simulink model "BFE_TestHarness"  (Simulink 8.6)
settings: Solver=FixedStepDiscrete  StartTime=0.0  StopTime=3  FixedStep=Ts  RelTol=1e-3
PreLoadFcn:
  | addpath('MBD_Tests')
  | 
  | load('Workspace\EnvVar.mat')
  | run('MBD_Tests\MBD_tests_init.m')
  | if exist('tl_preloadfcn','file'), tl_preloadfcn(gcs,402); end
PostLoadFcn:
  | if exist('tl_postloadfcn','file'), tl_postloadfcn(gcs,402); end
InitFcn:
  | if exist('tlds_init','file'), tlds_init(gcs); end
StartFcn:
  | if exist('tlds_start','file'), tlds_start(gcs); end
StopFcn:
  | if exist('tlds_stop','file'), tlds_stop(gcs); end
undefined symbols (not defined in the file): ddv, Ts, u2, u3, u4
libraries: tllib x11, simulink x8, LIB_TF_G_111 x2, LIB_TF_G_12_StepControl x2, LIB_TF_G_112 x1, LIB_TF_G_113 x1
(part 8 of 17)

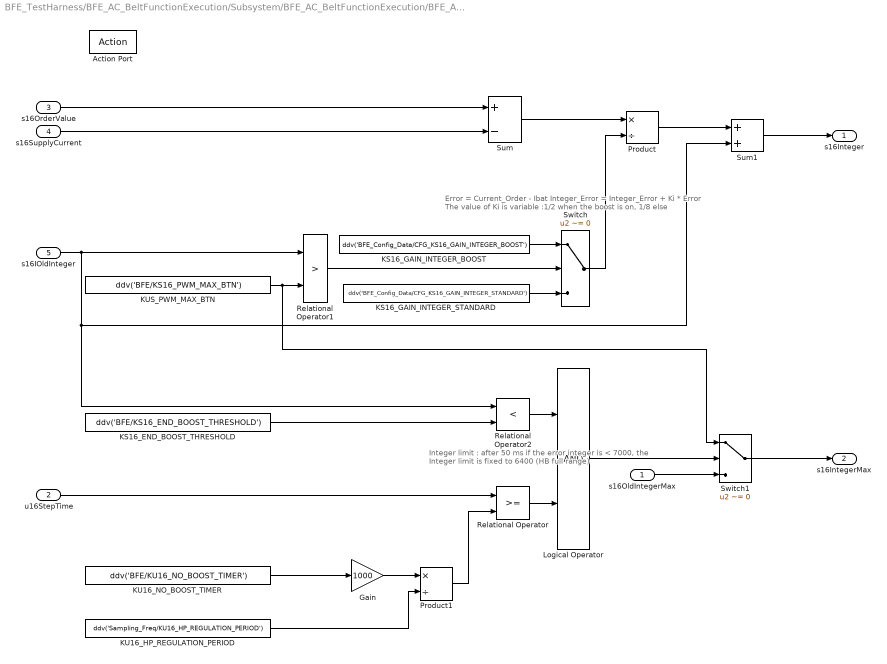
== system BFE_TestHarness/BFE_AC_BeltFunctionExecution/Subsystem/BFE_AC_BeltFunctionExecution/BFE_AC_BeltFunctionExecution/BFE_runExecuteHighPowerStep/HP feature activated/CurrentRegulation/PerformRegulation ==
  note: Error = Current_Order - Ibat
      | Integer_Error = Integer_Error + Ki * Error
      | The value of Ki is variable :1/2 when the boost is on, 1/8 else
  note: Integer limit : after 50 ms if the error integer is < 7000,
      | the Integer limit is fixed to 6400 (HB full range)
  s16OldIntegerMax : Inport  RequirementInfo={} %GIDa_4edf5c18_cfb4_4ed1_aec0_eafae2324e3a
  u16StepTime : Inport  RequirementInfo={} %GIDa_9a24bfd6_4e27_4306_b68d_5ae91b60016c  Port=2
  s16OrderValue : Inport  RequirementInfo={} %GIDa_b1229915_314b_4863_98e3_52cac1c2f91e  Port=3
  s16SupplyCurrent : Inport  RequirementInfo={} %GIDa_425d2a36_5fe9_4dc0_bde3_e336324c322d  Port=4
  s16IOldInteger : Inport  RequirementInfo={} %GIDa_71962a0c_10e9_4e80_9963_0f670b982034  Port=5
  Action Port : ActionPort  RequirementInfo={} %GIDa_15d562f7_52fc_451c_88e4_4cd9eea4c744  ActionType=else
  Gain : Gain  RequirementInfo={} %GIDa_ea57d22b_49e6_4b7f_ac29_28cc2dbba7b3  Gain=1000  OutDataTypeStr=uint16  mask(TL_Gain){data={'output',{'type','UInt16'},'date',735951.66844787041}}
      settings: CopyFcn=if exist('tl_reset_reviewflag','file')==2,tl_reset_reviewflag(gcbh);end  DeleteFcn=if exist('delete_tlblock','file')==2,delete_tlblock(gcbh);end  NameChangeFcn=if exist('rename_tlblock','file')==2,rename_tlblock(gcbh);end  OpenFcn=if exist('tl_open_blockdlg','file')==2,tl_open_blockdlg(gcbh);else,open_system(gcbh,'parameter');end
      mask Help: eval(['if exist(''tl_online_help'',''file'') == 2, tl_online_help(''Topic'',''TL_Gain''),else, web([''jar:file:///'',matlabroot,''/help/toolbox/simulink/help.jar!/slref/' lower(get_param(gcbh,'Blocktype')) '.html''], ''-helpbrowser''),end'])
      mask Display: plot([0, .9, 0],[.05, .5, .95])
  KS16_END_BOOST_THRESHOLD : Constant  RequirementInfo={} %GIDa_f3b0ac08_8bb7_400a_a265_f98ea3ab135f  Value=ddv('BFE/KS16_END_BOOST_THRESHOLD')  OutDataTypeStr=int16  mask(TL_Constant){data={'output',{'variable','BFE/KS16_END_BOOST_THRESHOLD'},'date',735951.66844737274}}
      settings: CopyFcn=if exist('tl_reset_reviewflag','file')==2,tl_reset_reviewflag(gcbh);end  DeleteFcn=if exist('delete_tlblock','file')==2,delete_tlblock(gcbh);end  NameChangeFcn=if exist('rename_tlblock','file')==2,rename_tlblock(gcbh);end  OpenFcn=if exist('tl_open_blockdlg','file')==2,tl_open_blockdlg(gcbh);else,open_system(gcbh,'parameter');end
      mask Help: eval(['if exist(''tl_online_help'',''file'') == 2, tl_online_help(''Topic'',''TL_Constant''),else, web([''jar:file:///'',matlabroot,''/help/toolbox/simulink/help.jar!/slref/' lower(get_param(gcbh,'Blocktype')) '.html''], ''-helpbrowser''),end'])
      mask Display: plot([-0.05, 1.05, NaN, -0.05, 1.05],[.01, .01, NaN, .99, .99])
  KS16_GAIN_INTEGER_BOOST : Constant  RequirementInfo={} %GIDa_006f4594_68bd_400b_90bf_0f2f50455285  Value=ddv('BFE_Config_Data/CFG_KS16_GAIN_INTEGER_BOOST')  OutDataTypeStr=int16  mask(TL_Constant){data={'output',{'variable','BFE_Config_Data/CFG_KS16_GAIN_INTEGER_BOOST'},'date',735951.6684470023}}
      settings: CopyFcn=if exist('tl_reset_reviewflag','file')==2,tl_reset_reviewflag(gcbh);end  DeleteFcn=if exist('delete_tlblock','file')==2,delete_tlblock(gcbh);end  NameChangeFcn=if exist('rename_tlblock','file')==2,rename_tlblock(gcbh);end  OpenFcn=if exist('tl_open_blockdlg','file')==2,tl_open_blockdlg(gcbh);else,open_system(gcbh,'parameter');end
      mask Help: eval(['if exist(''tl_online_help'',''file'') == 2, tl_online_help(''Topic'',''TL_Constant''),else, web([''jar:file:///'',matlabroot,''/help/toolbox/simulink/help.jar!/slref/' lower(get_param(gcbh,'Blocktype')) '.html''], ''-helpbrowser''),end'])
      mask Display: plot([-0.05, 1.05, NaN, -0.05, 1.05],[.01, .01, NaN, .99, .99])
  KS16_GAIN_INTEGER_STANDARD : Constant  RequirementInfo={} %GIDa_e385b7ef_ce71_4760_a7c3_e905cf32e7fa  Value=ddv('BFE_Config_Data/CFG_KS16_GAIN_INTEGER_STANDARD')  OutDataTypeStr=int16  mask(TL_Constant){data={'output',{'variable','BFE_Config_Data/CFG_KS16_GAIN_INTEGER_STANDARD'},'date',735951.66844662034}}
      settings: CopyFcn=if exist('tl_reset_reviewflag','file')==2,tl_reset_reviewflag(gcbh);end  DeleteFcn=if exist('delete_tlblock','file')==2,delete_tlblock(gcbh);end  NameChangeFcn=if exist('rename_tlblock','file')==2,rename_tlblock(gcbh);end  OpenFcn=if exist('tl_open_blockdlg','file')==2,tl_open_blockdlg(gcbh);else,open_system(gcbh,'parameter');end
      mask Help: eval(['if exist(''tl_online_help'',''file'') == 2, tl_online_help(''Topic'',''TL_Constant''),else, web([''jar:file:///'',matlabroot,''/help/toolbox/simulink/help.jar!/slref/' lower(get_param(gcbh,'Blocktype')) '.html''], ''-helpbrowser''),end'])
      mask Display: plot([-0.05, 1.05, NaN, -0.05, 1.05],[.01, .01, NaN, .99, .99])
  KU16_HP_REGULATION_PERIOD : Constant  RequirementInfo={} %GIDa_9a40dac7_f0ac_4b32_adfc_120258120a3a  Value=ddv('Sampling_Freq/KU16_HP_REGULATION_PERIOD')  mask(TL_Constant){data={'output',{'variable','Sampling_Freq/KU16_HP_REGULATION_PERIOD'},'date',735951.66844625003}}
      settings: CopyFcn=if exist('tl_reset_reviewflag','file')==2,tl_reset_reviewflag(gcbh);end  DeleteFcn=if exist('delete_tlblock','file')==2,delete_tlblock(gcbh);end  NameChangeFcn=if exist('rename_tlblock','file')==2,rename_tlblock(gcbh);end  OpenFcn=if exist('tl_open_blockdlg','file')==2,tl_open_blockdlg(gcbh);else,open_system(gcbh,'parameter');end
      mask Help: eval(['if exist(''tl_online_help'',''file'') == 2, tl_online_help(''Topic'',''TL_Constant''),else, web([''jar:file:///'',matlabroot,''/help/toolbox/simulink/help.jar!/slref/' lower(get_param(gcbh,'Blocktype')) '.html''], ''-helpbrowser''),end'])
      mask Display: plot([-0.05, 1.05, NaN, -0.05, 1.05],[.01, .01, NaN, .99, .99])
  KU16_NO_BOOST_TIMER : Constant  RequirementInfo={} %GIDa_e83b1f24_680d_46f7_a5ae_aeb7e7750aab  Value=ddv('BFE/KU16_NO_BOOST_TIMER')  OutDataTypeStr=uint16  mask(TL_Constant){data={'output',{'variable','BFE/KU16_NO_BOOST_TIMER'},'date',735951.66844587959}}
      settings: CopyFcn=if exist('tl_reset_reviewflag','file')==2,tl_reset_reviewflag(gcbh);end  DeleteFcn=if exist('delete_tlblock','file')==2,delete_tlblock(gcbh);end  NameChangeFcn=if exist('rename_tlblock','file')==2,rename_tlblock(gcbh);end  OpenFcn=if exist('tl_open_blockdlg','file')==2,tl_open_blockdlg(gcbh);else,open_system(gcbh,'parameter');end
      mask Help: eval(['if exist(''tl_online_help'',''file'') == 2, tl_online_help(''Topic'',''TL_Constant''),else, web([''jar:file:///'',matlabroot,''/help/toolbox/simulink/help.jar!/slref/' lower(get_param(gcbh,'Blocktype')) '.html''], ''-helpbrowser''),end'])
      mask Display: plot([-0.05, 1.05, NaN, -0.05, 1.05],[.01, .01, NaN, .99, .99])
  KUS_PWM_MAX_BTN : Constant  RequirementInfo={} %GIDa_d06a0857_79a9_48d4_af10_a27c76f3bd27  Value=ddv('BFE/KS16_PWM_MAX_BTN')  OutDataTypeStr=uint16  mask(TL_Constant){data={'output',{'variable','BFE/KS16_PWM_MAX_BTN'},'date',735951.66844550928}}
      settings: CopyFcn=if exist('tl_reset_reviewflag','file')==2,tl_reset_reviewflag(gcbh);end  DeleteFcn=if exist('delete_tlblock','file')==2,delete_tlblock(gcbh);end  NameChangeFcn=if exist('rename_tlblock','file')==2,rename_tlblock(gcbh);end  OpenFcn=if exist('tl_open_blockdlg','file')==2,tl_open_blockdlg(gcbh);else,open_system(gcbh,'parameter');end
      mask Help: eval(['if exist(''tl_online_help'',''file'') == 2, tl_online_help(''Topic'',''TL_Constant''),else, web([''jar:file:///'',matlabroot,''/help/toolbox/simulink/help.jar!/slref/' lower(get_param(gcbh,'Blocktype')) '.html''], ''-helpbrowser''),end'])
      mask Display: plot([-0.05, 1.05, NaN, -0.05, 1.05],[.01, .01, NaN, .99, .99])
  Logical Operator : Logic  RequirementInfo={} %GIDa_7b838156_8377_48ac_bbd6_b499fe2bfe99  AllPortsSameDT=off  OutDataTypeStr=boolean  mask(TL_LogicalOperator){data={'output',{'name','bNoMoreBoost'},'date',735951.66844513884}}
      settings: DeleteFcn=if exist('delete_tlblock','file')==2,delete_tlblock(gcbh);end  NameChangeFcn=if exist('rename_tlblock','file')==2,rename_tlblock(gcbh);end  OpenFcn=if exist('tl_open_blockdlg','file')==2,tl_open_blockdlg(gcbh);else,open_system(gcbh,'parameter');end
      mask Help: eval(['if exist(''tl_online_help'',''file'') == 2, tl_online_help(''Topic'',''TL_LogicalOperator''),else, web([''jar:file:///'',matlabroot,''/help/toolbox/simulink/help.jar!/slref/' lower(get_param(gcbh,'Blocktype')) '.html''], ''-helpbrowser''),end'])
      mask Display: plot([-0.05, 1.05, NaN, -0.05, 1.05],[.01, .01, NaN, .99, .99])
  Product : Product  RequirementInfo={} %GIDa_35ca37b1_04f3_43f1_ba53_a4e2a84b84d7  Inputs=*/  OutDataTypeStr=int16  RndMeth=Zero  mask(TL_Product){data={'output',{'name','s16CorrectedError'},'date',735951.66844486108}}
      settings: CopyFcn=if exist('tl_reset_reviewflag','file')==2,tl_reset_reviewflag(gcbh);end  DeleteFcn=if exist('delete_tlblock','file')==2,delete_tlblock(gcbh);end  NameChangeFcn=if exist('rename_tlblock','file')==2,rename_tlblock(gcbh);end  OpenFcn=if exist('tl_open_blockdlg','file')==2,tl_open_blockdlg(gcbh);else,open_system(gcbh,'parameter');end
      mask Help: eval(['if exist(''tl_online_help'',''file'') == 2, tl_online_help(''Topic'',''TL_Product''),else, web([''jar:file:///'',matlabroot,''/help/toolbox/simulink/help.jar!/slref/' lower(get_param(gcbh,'Blocktype')) '.html''], ''-helpbrowser''),end'])
      mask Display: plot([-0.05, 1.05, NaN, -0.05, 1.05],[.01, .01, NaN, .99, .99])
  Product1 : Product  RequirementInfo={} %GIDa_229b16f6_a871_42bd_ac54_44654e1e286c  Inputs=*/  RndMeth=Zero  mask(TL_Product){data={'output',{'name','u16StartBoostTimer','type','UInt16'},'date',735951.66844447912}}
      settings: CopyFcn=if exist('tl_reset_reviewflag','file')==2,tl_reset_reviewflag(gcbh);end  DeleteFcn=if exist('delete_tlblock','file')==2,delete_tlblock(gcbh);end  NameChangeFcn=if exist('rename_tlblock','file')==2,rename_tlblock(gcbh);end  OpenFcn=if exist('tl_open_blockdlg','file')==2,tl_open_blockdlg(gcbh);else,open_system(gcbh,'parameter');end
      mask Help: eval(['if exist(''tl_online_help'',''file'') == 2, tl_online_help(''Topic'',''TL_Product''),else, web([''jar:file:///'',matlabroot,''/help/toolbox/simulink/help.jar!/slref/' lower(get_param(gcbh,'Blocktype')) '.html''], ''-helpbrowser''),end'])
      mask Display: plot([-0.05, 1.05, NaN, -0.05, 1.05],[.01, .01, NaN, .99, .99])
  Relational Operator : RelationalOperator  RequirementInfo={} %GIDa_fc758f8d_8d88_4bb2_a782_7020b49923fd  OutDataTypeStr=boolean  mask(TL_RelationalOperator){data={'output',{'name','bIsStartBoostPeriod'},'date',735951.66844412033}}
      settings: DeleteFcn=if exist('delete_tlblock','file')==2,delete_tlblock(gcbh);end  NameChangeFcn=if exist('rename_tlblock','file')==2,rename_tlblock(gcbh);end  OpenFcn=if exist('tl_open_blockdlg','file')==2,tl_open_blockdlg(gcbh);else,open_system(gcbh,'parameter');end
      mask Help: eval(['if exist(''tl_online_help'',''file'') == 2, tl_online_help(''Topic'',''TL_RelationalOperator''),else, web([''jar:file:///'',matlabroot,''/help/toolbox/simulink/help.jar!/slref/' lower(get_param(gcbh,'Blocktype')) '.html''], ''-helpbrowser''),end'])
      mask Display: plot([-0.05, 1.05, NaN, -0.05, 1.05],[.01, .01, NaN, .99, .99])
  Relational Operator1 : RelationalOperator  RequirementInfo={} %GIDa_b74c9104_faae_464c_abe5_108504633b0e  Operator=>  OutDataTypeStr=boolean  mask(TL_RelationalOperator){data={'output',{'name','bIsBoostOn'},'date',735951.66844387737}}
      settings: DeleteFcn=if exist('delete_tlblock','file')==2,delete_tlblock(gcbh);end  NameChangeFcn=if exist('rename_tlblock','file')==2,rename_tlblock(gcbh);end  OpenFcn=if exist('tl_open_blockdlg','file')==2,tl_open_blockdlg(gcbh);else,open_system(gcbh,'parameter');end
      mask Help: eval(['if exist(''tl_online_help'',''file'') == 2, tl_online_help(''Topic'',''TL_RelationalOperator''),else, web([''jar:file:///'',matlabroot,''/help/toolbox/simulink/help.jar!/slref/' lower(get_param(gcbh,'Blocktype')) '.html''], ''-helpbrowser''),end'])
      mask Display: plot([-0.05, 1.05, NaN, -0.05, 1.05],[.01, .01, NaN, .99, .99])
  Relational Operator2 : RelationalOperator  RequirementInfo={} %GIDa_ad16e991_7f4e_4203_a22d_63b6bdc27e5f  Operator=<  OutDataTypeStr=boolean  mask(TL_RelationalOperator){data={'output',{'name','bEndOfBoost'},'date',735951.66844362265}}
      settings: DeleteFcn=if exist('delete_tlblock','file')==2,delete_tlblock(gcbh);end  NameChangeFcn=if exist('rename_tlblock','file')==2,rename_tlblock(gcbh);end  OpenFcn=if exist('tl_open_blockdlg','file')==2,tl_open_blockdlg(gcbh);else,open_system(gcbh,'parameter');end
      mask Help: eval(['if exist(''tl_online_help'',''file'') == 2, tl_online_help(''Topic'',''TL_RelationalOperator''),else, web([''jar:file:///'',matlabroot,''/help/toolbox/simulink/help.jar!/slref/' lower(get_param(gcbh,'Blocktype')) '.html''], ''-helpbrowser''),end'])
      mask Display: plot([-0.05, 1.05, NaN, -0.05, 1.05],[.01, .01, NaN, .99, .99])
  Sum : Sum  RequirementInfo={} %GIDa_536419a0_529a_4f87_8818_e3cf6708e55d  Inputs=+-  mask(TL_Sum){data={'output',{'name','s16CurrentError'},'date',735951.66844335652}}
      settings: CopyFcn=if exist('tl_reset_reviewflag','file')==2,tl_reset_reviewflag(gcbh);end  DeleteFcn=if exist('delete_tlblock','file')==2,delete_tlblock(gcbh);end  NameChangeFcn=if exist('rename_tlblock','file')==2,rename_tlblock(gcbh);end  OpenFcn=if exist('tl_open_blockdlg','file')==2,tl_open_blockdlg(gcbh);else,open_system(gcbh,'parameter');end
      mask Help: eval(['if exist(''tl_online_help'',''file'') == 2, tl_online_help(''Topic'',''TL_Sum''),else, web([''jar:file:///'',matlabroot,''/help/toolbox/simulink/help.jar!/slref/' lower(get_param(gcbh,'Blocktype')) '.html''], ''-helpbrowser''),end'])
      mask Display: plot([-0.05, 1.05, NaN, -0.05, 1.05],[.01, .01, NaN, .99, .99])
  Sum1 : Sum  RequirementInfo={} %GIDa_fd09ff90_0e60_4170_8070_f34ee1cc6f7e  mask(TL_Sum){data={'output',{'name','s16IntegerError'},'date',735951.66844298609}}
      settings: CopyFcn=if exist('tl_reset_reviewflag','file')==2,tl_reset_reviewflag(gcbh);end  DeleteFcn=if exist('delete_tlblock','file')==2,delete_tlblock(gcbh);end  NameChangeFcn=if exist('rename_tlblock','file')==2,rename_tlblock(gcbh);end  OpenFcn=if exist('tl_open_blockdlg','file')==2,tl_open_blockdlg(gcbh);else,open_system(gcbh,'parameter');end
      mask Help: eval(['if exist(''tl_online_help'',''file'') == 2, tl_online_help(''Topic'',''TL_Sum''),else, web([''jar:file:///'',matlabroot,''/help/toolbox/simulink/help.jar!/slref/' lower(get_param(gcbh,'Blocktype')) '.html''], ''-helpbrowser''),end'])
      mask Display: plot([-0.05, 1.05, NaN, -0.05, 1.05],[.01, .01, NaN, .99, .99])
  Switch : Switch  RequirementInfo={} %GIDa_afeac32e_f260_4c89_8c9f_a864b6e54b1d  Criteria=u2 ~= 0  Threshold=ddv('BFE/KS16_PWM_MAX_BTN')  mask(TL_Switch){data={'date',735951.66844259261}}
      settings: CopyFcn=if exist('tl_reset_reviewflag','file')==2,tl_reset_reviewflag(gcbh);end  DeleteFcn=if exist('delete_tlblock','file')==2,delete_tlblock(gcbh);end  NameChangeFcn=if exist('rename_tlblock','file')==2,rename_tlblock(gcbh);end  OpenFcn=if exist('tl_open_blockdlg','file')==2,tl_open_blockdlg(gcbh);else,open_system(gcbh,'parameter');end
      mask Help: eval(['if exist(''tl_online_help'',''file'') == 2, tl_online_help(''Topic'',''TL_Switch''),else, web([''jar:file:///'',matlabroot,''/help/toolbox/simulink/help.jar!/slref/' lower(get_param(gcbh,'Blocktype')) '.html''], ''-helpbrowser''),end'])
      mask Display: plot([-0.05, 1.05, NaN, -0.05, 1.05],[.01, .01, NaN, .99, .99])
  Switch1 : Switch  RequirementInfo={} %GIDa_14b28a10_4214_42aa_bdf6_ce99bb3abf67  Criteria=u2 ~= 0  OutDataTypeStr=int16  mask(TL_Switch){data={'date',735951.66844207176}}
      settings: CopyFcn=if exist('tl_reset_reviewflag','file')==2,tl_reset_reviewflag(gcbh);end  DeleteFcn=if exist('delete_tlblock','file')==2,delete_tlblock(gcbh);end  NameChangeFcn=if exist('rename_tlblock','file')==2,rename_tlblock(gcbh);end  OpenFcn=if exist('tl_open_blockdlg','file')==2,tl_open_blockdlg(gcbh);else,open_system(gcbh,'parameter');end
      mask Help: eval(['if exist(''tl_online_help'',''file'') == 2, tl_online_help(''Topic'',''TL_Switch''),else, web([''jar:file:///'',matlabroot,''/help/toolbox/simulink/help.jar!/slref/' lower(get_param(gcbh,'Blocktype')) '.html''], ''-helpbrowser''),end'])
      mask Display: plot([-0.05, 1.05, NaN, -0.05, 1.05],[.01, .01, NaN, .99, .99])
  s16Integer : Outport  RequirementInfo={} %GIDa_26c1c79d_22c0_410b_b45a_f21ec8537878  OutDataTypeStr=int16  InitialOutput=0
  s16IntegerMax : Outport  RequirementInfo={} %GIDa_934635ec_890b_4177_a190_582d0e969087  Port=2  OutDataTypeStr=int16  InitialOutput=0
  wires:
  Sum/1 -> Product/1
  Product/1 -> Sum1/1
  s16OrderValue/1 -> Sum/1
  s16SupplyCurrent/1 -> Sum/2
  Switch/1 -> Product/2
  s16IOldInteger/1 -> Relational Operator1/1, Sum1/2, Relational Operator2/1
  KS16_GAIN_INTEGER_BOOST/1 -> Switch/1
  KS16_GAIN_INTEGER_STANDARD/1 -> Switch/3
  KUS_PWM_MAX_BTN/1 -> Relational Operator1/2, Switch1/1
  Relational Operator1/1 -> Switch/2
  Sum1/1 -> s16Integer/1
  KU16_HP_REGULATION_PERIOD/1 -> Product1/2
  Gain/1 -> Product1/1
  Relational Operator/1 -> Logical Operator/2
  Logical Operator/1 -> Switch1/2
  KS16_END_BOOST_THRESHOLD/1 -> Relational Operator2/2
  Relational Operator2/1 -> Logical Operator/1
  u16StepTime/1 -> Relational Operator/1
  Product1/1 -> Relational Operator/2
  KU16_NO_BOOST_TIMER/1 -> Gain/1
  s16OldIntegerMax/1 -> Switch1/3
  Switch1/1 -> s16IntegerMax/1

== system BFE_TestHarness/BFE_AC_BeltFunctionExecution/Subsystem/BFE_AC_BeltFunctionExecution/BFE_AC_BeltFunctionExecution/BFE_runExecuteHighPowerStep/HP feature activated/CurrentRegulation/SlowBoostDecrease ==
  note: The value of the duty cycle on the boost is decreased softly before the end of the step, in order to avoid to fall to 0 too quickly (risk for the transistor if the boost is shut down suddenly)
  s16OldIntegerMax : Inport  RequirementInfo={} %GIDa_89c0824a_6372_451d_84e5_84db3e0a11ef
  s16IOldInteger : Inport  RequirementInfo={} %GIDa_a80bd93b_fecd_4610_8ce4_dd930f94cd42  Port=2
  Action Port : ActionPort  RequirementInfo={} %GIDa_e3d5b2f1_3f0f_4458_8047_9dfcc3d73cfb  ActionType=then
  Constant1 : Constant  RequirementInfo={} %GIDa_2321a1d8_90d8_4230_9977_c3174d88ff39  Value=ddv('BFE/KS16_PWM_MAX_BTN')  OutDataTypeStr=uint16  mask(TL_Constant){data={'output',{'variable','BFE/KS16_PWM_MAX_BTN'},'date',735951.66844144673}}
      settings: CopyFcn=if exist('tl_reset_reviewflag','file')==2,tl_reset_reviewflag(gcbh);end  DeleteFcn=if exist('delete_tlblock','file')==2,delete_tlblock(gcbh);end  NameChangeFcn=if exist('rename_tlblock','file')==2,rename_tlblock(gcbh);end  OpenFcn=if exist('tl_open_blockdlg','file')==2,tl_open_blockdlg(gcbh);else,open_system(gcbh,'parameter');end
      mask Help: eval(['if exist(''tl_online_help'',''file'') == 2, tl_online_help(''Topic'',''TL_Constant''),else, web([''jar:file:///'',matlabroot,''/help/toolbox/simulink/help.jar!/slref/' lower(get_param(gcbh,'Blocktype')) '.html''], ''-helpbrowser''),end'])
      mask Display: plot([-0.05, 1.05, NaN, -0.05, 1.05],[.01, .01, NaN, .99, .99])
  Constant2 : Constant  RequirementInfo={} %GIDa_51b21838_217e_4208_8f63_f35d4216c2d7  Value=ddv('BFE_Config_Data/KUS_STEP_DECREASE_PWMBOOST')  OutDataTypeStr=uint16  mask(TL_Constant){data={'output',{'variable','BFE_Config_Data/KUS_STEP_DECREASE_PWMBOOST'},'date',735951.66844108794}}
      settings: CopyFcn=if exist('tl_reset_reviewflag','file')==2,tl_reset_reviewflag(gcbh);end  DeleteFcn=if exist('delete_tlblock','file')==2,delete_tlblock(gcbh);end  NameChangeFcn=if exist('rename_tlblock','file')==2,rename_tlblock(gcbh);end  OpenFcn=if exist('tl_open_blockdlg','file')==2,tl_open_blockdlg(gcbh);else,open_system(gcbh,'parameter');end
      mask Help: eval(['if exist(''tl_online_help'',''file'') == 2, tl_online_help(''Topic'',''TL_Constant''),else, web([''jar:file:///'',matlabroot,''/help/toolbox/simulink/help.jar!/slref/' lower(get_param(gcbh,'Blocktype')) '.html''], ''-helpbrowser''),end'])
      mask Display: plot([-0.05, 1.05, NaN, -0.05, 1.05],[.01, .01, NaN, .99, .99])
  Constant3 : Constant  RequirementInfo={} %GIDa_f3dc36c4_dddd_49b7_97d1_20aa0210a17f  Value=ddv('BFE/KS16_PWM_MAX_BTN')  OutDataTypeStr=uint16  mask(TL_Constant){data={'output',{'variable','BFE/KS16_PWM_MAX_BTN'},'date',735951.66844071762}}
      settings: CopyFcn=if exist('tl_reset_reviewflag','file')==2,tl_reset_reviewflag(gcbh);end  DeleteFcn=if exist('delete_tlblock','file')==2,delete_tlblock(gcbh);end  NameChangeFcn=if exist('rename_tlblock','file')==2,rename_tlblock(gcbh);end  OpenFcn=if exist('tl_open_blockdlg','file')==2,tl_open_blockdlg(gcbh);else,open_system(gcbh,'parameter');end
      mask Help: eval(['if exist(''tl_online_help'',''file'') == 2, tl_online_help(''Topic'',''TL_Constant''),else, web([''jar:file:///'',matlabroot,''/help/toolbox/simulink/help.jar!/slref/' lower(get_param(gcbh,'Blocktype')) '.html''], ''-helpbrowser''),end'])
      mask Display: plot([-0.05, 1.05, NaN, -0.05, 1.05],[.01, .01, NaN, .99, .99])
  Relational Operator1 : RelationalOperator  RequirementInfo={} %GIDa_5308457e_821a_4f16_a7d9_22de4725e4a4  Operator=>  OutDataTypeStr=boolean  mask(TL_RelationalOperator){data={'output',{'name','bIsStillBoost'},'date',735951.66844034719}}
      settings: DeleteFcn=if exist('delete_tlblock','file')==2,delete_tlblock(gcbh);end  NameChangeFcn=if exist('rename_tlblock','file')==2,rename_tlblock(gcbh);end  OpenFcn=if exist('tl_open_blockdlg','file')==2,tl_open_blockdlg(gcbh);else,open_system(gcbh,'parameter');end
      mask Help: eval(['if exist(''tl_online_help'',''file'') == 2, tl_online_help(''Topic'',''TL_RelationalOperator''),else, web([''jar:file:///'',matlabroot,''/help/toolbox/simulink/help.jar!/slref/' lower(get_param(gcbh,'Blocktype')) '.html''], ''-helpbrowser''),end'])
      mask Display: plot([-0.05, 1.05, NaN, -0.05, 1.05],[.01, .01, NaN, .99, .99])
  Relational Operator2 : RelationalOperator  RequirementInfo={} %GIDa_81850835_e86c_4d48_bd9c_8a51da59653e  Operator=<  OutDataTypeStr=boolean  mask(TL_RelationalOperator){data={'output',{'name','bIsIntegerMaxTooLow'},'date',735951.66844010411}}
      settings: DeleteFcn=if exist('delete_tlblock','file')==2,delete_tlblock(gcbh);end  NameChangeFcn=if exist('rename_tlblock','file')==2,rename_tlblock(gcbh);end  OpenFcn=if exist('tl_open_blockdlg','file')==2,tl_open_blockdlg(gcbh);else,open_system(gcbh,'parameter');end
      mask Help: eval(['if exist(''tl_online_help'',''file'') == 2, tl_online_help(''Topic'',''TL_RelationalOperator''),else, web([''jar:file:///'',matlabroot,''/help/toolbox/simulink/help.jar!/slref/' lower(get_param(gcbh,'Blocktype')) '.html''], ''-helpbrowser''),end'])
      mask Display: plot([-0.05, 1.05, NaN, -0.05, 1.05],[.01, .01, NaN, .99, .99])
  Sum : Sum  RequirementInfo={} %GIDa_6bddf89d_4df6_4e26_9efd_7c057f48ffb3  Inputs=+-  AccumDataTypeStr=int16  OutDataTypeStr=int16  mask(TL_Sum){data={'output',{'name','s16_IntegerMaxReduced'},'date',735951.66843983799}}
      settings: CopyFcn=if exist('tl_reset_reviewflag','file')==2,tl_reset_reviewflag(gcbh);end  DeleteFcn=if exist('delete_tlblock','file')==2,delete_tlblock(gcbh);end  NameChangeFcn=if exist('rename_tlblock','file')==2,rename_tlblock(gcbh);end  OpenFcn=if exist('tl_open_blockdlg','file')==2,tl_open_blockdlg(gcbh);else,open_system(gcbh,'parameter');end
      mask Help: eval(['if exist(''tl_online_help'',''file'') == 2, tl_online_help(''Topic'',''TL_Sum''),else, web([''jar:file:///'',matlabroot,''/help/toolbox/simulink/help.jar!/slref/' lower(get_param(gcbh,'Blocktype')) '.html''], ''-helpbrowser''),end'])
      mask Display: plot([-0.05, 1.05, NaN, -0.05, 1.05],[.01, .01, NaN, .99, .99])
  Switch1 : Switch  RequirementInfo={} %GIDa_6864e359_53bc_4108_bf49_734d67f89f18  Criteria=u2 ~= 0  OutDataTypeStr=int16  mask(TL_Switch){data={'output',{'name','s16_IntegerMaxSwitch'},'date',735951.66843945603}}
      settings: CopyFcn=if exist('tl_reset_reviewflag','file')==2,tl_reset_reviewflag(gcbh);end  DeleteFcn=if exist('delete_tlblock','file')==2,delete_tlblock(gcbh);end  NameChangeFcn=if exist('rename_tlblock','file')==2,rename_tlblock(gcbh);end  OpenFcn=if exist('tl_open_blockdlg','file')==2,tl_open_blockdlg(gcbh);else,open_system(gcbh,'parameter');end
      mask Help: eval(['if exist(''tl_online_help'',''file'') == 2, tl_online_help(''Topic'',''TL_Switch''),else, web([''jar:file:///'',matlabroot,''/help/toolbox/simulink/help.jar!/slref/' lower(get_param(gcbh,'Blocktype')) '.html''], ''-helpbrowser''),end'])
      mask Display: plot([-0.05, 1.05, NaN, -0.05, 1.05],[.01, .01, NaN, .99, .99])
  Switch2 : Switch  RequirementInfo={} %GIDa_01c4b7fd_9c0b_4706_aa1b_f1d3a4d3cf2b  Criteria=u2 ~= 0  OutDataTypeStr=int16  mask(TL_Switch){data={'output',{'name','s16IntegerMaxDecreased'},'date',735951.66843890049}}
      settings: CopyFcn=if exist('tl_reset_reviewflag','file')==2,tl_reset_reviewflag(gcbh);end  DeleteFcn=if exist('delete_tlblock','file')==2,delete_tlblock(gcbh);end  NameChangeFcn=if exist('rename_tlblock','file')==2,rename_tlblock(gcbh);end  OpenFcn=if exist('tl_open_blockdlg','file')==2,tl_open_blockdlg(gcbh);else,open_system(gcbh,'parameter');end
      mask Help: eval(['if exist(''tl_online_help'',''file'') == 2, tl_online_help(''Topic'',''TL_Switch''),else, web([''jar:file:///'',matlabroot,''/help/toolbox/simulink/help.jar!/slref/' lower(get_param(gcbh,'Blocktype')) '.html''], ''-helpbrowser''),end'])
      mask Display: plot([-0.05, 1.05, NaN, -0.05, 1.05],[.01, .01, NaN, .99, .99])
  s16Integer : Outport  RequirementInfo={} %GIDa_28f7edc3_ad42_4a06_b0bf_5d9c453a176c  InitialOutput=0
  sIntegerMax : Outport  RequirementInfo={} %GIDa_ef74e895_f434_406e_9a43_d385bb5283ca  Port=2  InitialOutput=0
  wires:
  s16OldIntegerMax/1 -> Relational Operator1/1, Sum/1, Switch1/3
  Relational Operator1/1 -> Switch1/2
  Constant2/1 -> Sum/2
  Sum/1 -> Switch1/1
  Switch1/1 -> Relational Operator2/1, Switch2/3
  Relational Operator2/1 -> Switch2/2
  Constant1/1 -> Relational Operator1/2
  Switch2/1 -> sIntegerMax/1
  Constant3/1 -> Relational Operator2/2, Switch2/1
  s16IOldInteger/1 -> s16Integer/1

== system BFE_TestHarness/BFE_AC_BeltFunctionExecution/Subsystem/BFE_AC_BeltFunctionExecution/BFE_AC_BeltFunctionExecution/BFE_runExecuteHighPowerStep/HP feature activated/CurrentRegulation/SupplyCurrent ==
  note: Calculation of the supply current ==> Resolution : 1A = 100 LSB
  MotorSign : Inport  RequirementInfo={} %GIDa_235cb0d6_8a0d_4f13_a1dd_acee295532cf
  ReadMotorCurrentInmA : Inport  RequirementInfo={} %GIDa_3e322c1e_e84c_45a7_8654_e9f56cea4a63  Port=2
  s16IOldInteger : Inport  RequirementInfo={} %GIDa_62b53cb4_65a0_4d26_a34a_f19732a1a2dd  Port=3
  bIsNewCycle : Inport  RequirementInfo={} %GIDa_0644e3ee_3697_415b_8241_25c4ee681db3  Port=4
  Drift_Compensation : Subsystem  RequirementInfo={} %GIDa_0756cf7e_cdb9_4179_9502_415c10322b41
  KUS_PWM_MAX_BTN : Constant  RequirementInfo={} %GIDa_9393248a_cd6e_483b_a030_678e36f1db23  Value=ddv('BFE/KS16_PWM_MAX_BTN')  OutDataTypeStr=uint16  mask(TL_Constant){data={'output',{'variable','BFE/KS16_PWM_MAX_BTN'},'date',735951.66842144681}}
      settings: CopyFcn=if exist('tl_reset_reviewflag','file')==2,tl_reset_reviewflag(gcbh);end  DeleteFcn=if exist('delete_tlblock','file')==2,delete_tlblock(gcbh);end  NameChangeFcn=if exist('rename_tlblock','file')==2,rename_tlblock(gcbh);end  OpenFcn=if exist('tl_open_blockdlg','file')==2,tl_open_blockdlg(gcbh);else,open_system(gcbh,'parameter');end
      mask Help: eval(['if exist(''tl_online_help'',''file'') == 2, tl_online_help(''Topic'',''TL_Constant''),else, web([''jar:file:///'',matlabroot,''/help/toolbox/simulink/help.jar!/slref/' lower(get_param(gcbh,'Blocktype')) '.html''], ''-helpbrowser''),end'])
      mask Display: plot([-0.05, 1.05, NaN, -0.05, 1.05],[.01, .01, NaN, .99, .99])
  Product1 : Product  RequirementInfo={} %GIDa_fc10b4b2_9c2a_4496_9594_2856e9fc16ea  Inputs=**  OutDataTypeStr=int32  RndMeth=Zero  mask(TL_Product){data={'output',{'type','Int32'},'date',735951.66842104169}}
      settings: CopyFcn=if exist('tl_reset_reviewflag','file')==2,tl_reset_reviewflag(gcbh);end  DeleteFcn=if exist('delete_tlblock','file')==2,delete_tlblock(gcbh);end  NameChangeFcn=if exist('rename_tlblock','file')==2,rename_tlblock(gcbh);end  OpenFcn=if exist('tl_open_blockdlg','file')==2,tl_open_blockdlg(gcbh);else,open_system(gcbh,'parameter');end
      mask Help: eval(['if exist(''tl_online_help'',''file'') == 2, tl_online_help(''Topic'',''TL_Product''),else, web([''jar:file:///'',matlabroot,''/help/toolbox/simulink/help.jar!/slref/' lower(get_param(gcbh,'Blocktype')) '.html''], ''-helpbrowser''),end'])
      mask Display: plot([-0.05, 1.05, NaN, -0.05, 1.05],[.01, .01, NaN, .99, .99])
  Product2 : Product  RequirementInfo={} %GIDa_5f6df54c_aaa4_4402_87ee_6d5ed2597bd5  Inputs=/*  OutDataTypeStr=int16  RndMeth=Zero  mask(TL_Product){data={'output',{'name','s16SupplyCurrent'},'date',735951.66842068289}}
      settings: CopyFcn=if exist('tl_reset_reviewflag','file')==2,tl_reset_reviewflag(gcbh);end  DeleteFcn=if exist('delete_tlblock','file')==2,delete_tlblock(gcbh);end  NameChangeFcn=if exist('rename_tlblock','file')==2,rename_tlblock(gcbh);end  OpenFcn=if exist('tl_open_blockdlg','file')==2,tl_open_blockdlg(gcbh);else,open_system(gcbh,'parameter');end
      mask Help: eval(['if exist(''tl_online_help'',''file'') == 2, tl_online_help(''Topic'',''TL_Product''),else, web([''jar:file:///'',matlabroot,''/help/toolbox/simulink/help.jar!/slref/' lower(get_param(gcbh,'Blocktype')) '.html''], ''-helpbrowser''),end'])
      mask Display: plot([-0.05, 1.05, NaN, -0.05, 1.05],[.01, .01, NaN, .99, .99])
  RescaleMotorMeasure : Subsystem  RequirementInfo={} %GIDa_a7e14cc9_3a8b_42f0_9dbe_0efff0e1864d
  s16SupplyCurrent : Outport  RequirementInfo={} %GIDa_f3c1e677_a485_49ce_b334_758196328594  OutDataTypeStr=int16  InitialOutput=0
  wires:
  MotorSign/1 -> RescaleMotorMeasure/1(MotorSigned)
  ReadMotorCurrentInmA/1 -> RescaleMotorMeasure/2(MotorUnsigned)
  Product1/1 -> Product2/2
  KUS_PWM_MAX_BTN/1 -> Product2/1
  s16IOldInteger/1 -> Product1/2
  Product2/1 -> s16SupplyCurrent/1
  bIsNewCycle/1 -> Drift_Compensation/2(bIsNewCycle)
  RescaleMotorMeasure/1(s16MotorCurrent) -> Drift_Compensation/1(s16MotorCurrent)
  Drift_Compensation/1(s16CorrectedMotorCurrent) -> Product1/1

== system BFE_TestHarness/BFE_AC_BeltFunctionExecution/Subsystem/BFE_AC_BeltFunctionExecution/BFE_AC_BeltFunctionExecution/BFE_runExecuteStandardSteps/ExecuteStandardSteps/Mange Power Stage consign update/Call PAL service to update the PWM ==
  In1 : Inport
  u8MotorStageStatus : Inport  Port=2
  Trigger : TriggerPort  TriggerType=function-call
  Apply power order : Subsystem  RequirementInfo={} %GIDa_8ebf7532_74cd_4bc0_846f_b603aef40d94  TreatAsAtomicUnit=on
  If : If  RequirementInfo={} %GIDa_87fbd21d_f512_4ba6_b659_e75628c03e7c  IfExpression=u1  ShowElse=off
  Motor stage nominal mode : Constant  RequirementInfo={} %GIDa_e3308c27_1114_44ed_9e0f_23acc9446faf  Value=ddv('RTE_Define/KU8_MOTOR_STAGE_ACTIVATION')  OutDataTypeStr=uint8  mask(TL_Constant){data={'output',{'variable','RTE_Define/KU8_MOTOR_STAGE_ACTIVATION'},'date',735951.66839996527}}
      settings: CopyFcn=if exist('tl_reset_reviewflag','file')==2,tl_reset_reviewflag(gcbh);end  DeleteFcn=if exist('delete_tlblock','file')==2,delete_tlblock(gcbh);end  NameChangeFcn=if exist('rename_tlblock','file')==2,rename_tlblock(gcbh);end  OpenFcn=if exist('tl_open_blockdlg','file')==2,tl_open_blockdlg(gcbh);else,open_system(gcbh,'parameter');end
      mask Help: eval(['if exist(''tl_online_help'',''file'') == 2, tl_online_help(''Topic'',''TL_Constant''),else, web([''jar:file:///'',matlabroot,''/help/toolbox/simulink/help.jar!/slref/' lower(get_param(gcbh,'Blocktype')) '.html''], ''-helpbrowser''),end'])
      mask Display: plot([-0.05, 1.05, NaN, -0.05, 1.05],[.01, .01, NaN, .99, .99])
  Relational Operator1 : RelationalOperator  Operator===  OutDataTypeStr=boolean  mask(TL_RelationalOperator){data={'date',735951.66839959496}}
      settings: DeleteFcn=if exist('delete_tlblock','file')==2,delete_tlblock(gcbh);end  NameChangeFcn=if exist('rename_tlblock','file')==2,rename_tlblock(gcbh);end  OpenFcn=if exist('tl_open_blockdlg','file')==2,tl_open_blockdlg(gcbh);else,open_system(gcbh,'parameter');end
      mask Help: eval(['if exist(''tl_online_help'',''file'') == 2, tl_online_help(''Topic'',''TL_RelationalOperator''),else, web([''jar:file:///'',matlabroot,''/help/toolbox/simulink/help.jar!/slref/' lower(get_param(gcbh,'Blocktype')) '.html''], ''-helpbrowser''),end'])
      mask Display: plot([-0.05, 1.05, NaN, -0.05, 1.05],[.01, .01, NaN, .99, .99])
  SSCP_pclMotorPowerOrder_SetPowerOrder : Outport
  s16MotorPowerOrder1 : Outport  Port=2
  wires:
  Motor stage nominal mode/1 -> Relational Operator1/1
  u8MotorStageStatus/1 -> Relational Operator1/2
  Relational Operator1/1 -> If/1
  Apply power order/1(SSCP_pclMotorPowerOrder_SetPowerOrder) -> SSCP_pclMotorPowerOrder_SetPowerOrder/1
  Apply power order/2(s16MotorPowerOrder1) -> s16MotorPowerOrder1/1
  In1/1 -> Apply power order/1(In1)  "s16MotorPowerOrder"
  If/1 -> Apply power order/Action

== system BFE_TestHarness/BFE_AC_BeltFunctionExecution/Subsystem/BFE_AC_BeltFunctionExecution/BFE_AC_BeltFunctionExecution/BFE_runExecuteStandardSteps/ExecuteStandardSteps/Mange Power Stage consign update/Resume ISR ==
  Trigger : TriggerPort  TriggerType=function-call
  Function : tllib/Function  data={'stepfunctionname','BFE_ExitCriticalSection','stepfunctionclass','EXTERN_FCN_CRITICAL_SECTION','restartfunctionname','RESTART_$B','initfunctionname','INIT_$B','termfunctionname','TERM_$B','date',735951.66833726852}  displayString=FUNCTION

== system BFE_TestHarness/BFE_AC_BeltFunctionExecution/Subsystem/BFE_AC_BeltFunctionExecution/BFE_AC_BeltFunctionExecution/BFE_runExecuteStandardSteps/ExecuteStandardSteps/Mange Power Stage consign update/Suspend ISR ==
  Trigger : TriggerPort  TriggerType=function-call
  Function : tllib/Function  data={'stepfunctionname','BFE_EnterCriticalSection','stepfunctionclass','EXTERN_FCN_CRITICAL_SECTION','restartfunctionname','RESTART_$B','initfunctionname','INIT_$B','termfunctionname','TERM_$B','date',735951.6683359259}  displayString=FUNCTION

== system BFE_TestHarness/BFE_AC_BeltFunctionExecution/Subsystem/BFE_AC_BeltFunctionExecution/BFE_AC_BeltFunctionExecution/BFE_runExecuteStandardSteps/ExecuteStandardSteps/SubsystemConvertOrderToMotorPower/Current_Regulation ==
  s32OrderToApply : Inport  RequirementInfo={} %GIDa_d7d43be5_3d35_4292_9174_5ee86be99e37
  u32MeasuredCurrent : Inport  RequirementInfo={} %GIDa_e2d4d881_0879_43fd_bcf0_fa1ec83e080f  Port=2
  s16OldPWM : Inport  RequirementInfo={} %GIDa_5f1e8450_433f_4318_beaf_9f47ba9afc79  Port=3
  u16BatteryVoltage : Inport  RequirementInfo={} %GIDa_8ed1e462_0d62_4079_8f5b_7d6503182d3c  Port=4
  bIsNewCycle : Inport  RequirementInfo={} %GIDa_08d3a65a_5879_45cd_8fe5_861edcc2dfdb  Port=5
  bIsPIDMotor : Inport  RequirementInfo={} %GIDa_37cf555f_5b7a_4e0a_85e9_4be93aa7c880  Port=6
  bIsPIDSupply : Inport  RequirementInfo={} %GIDa_c0823080_1ae4_44e3_b51e_77394796cf29  Port=7
  s32OldErrorInteger : Inport  RequirementInfo={} %GIDa_100cbe15_2bd7_4260_9333_3d9281fd01d0  Port=8
  bIsNewStepBegin : Inport  RequirementInfo={} %GIDa_b0d04fff_4020_42a9_b181_05ec63d3b4df  Port=9
  Action Port : ActionPort  RequirementInfo={} %GIDa_44edb1af_ff1c_497b_b2e8_fe5d8fa7987d  ActionType=case
  Gain : Gain  RequirementInfo={} %GIDa_70ee22be_249b_4a74_a84d_4a0ed2c559b7  OutDataTypeStr=int16  mask(TL_Gain){data={'date',735951.66839861113}}
      settings: CopyFcn=if exist('tl_reset_reviewflag','file')==2,tl_reset_reviewflag(gcbh);end  DeleteFcn=if exist('delete_tlblock','file')==2,delete_tlblock(gcbh);end  NameChangeFcn=if exist('rename_tlblock','file')==2,rename_tlblock(gcbh);end  OpenFcn=if exist('tl_open_blockdlg','file')==2,tl_open_blockdlg(gcbh);else,open_system(gcbh,'parameter');end
      mask Help: eval(['if exist(''tl_online_help'',''file'') == 2, tl_online_help(''Topic'',''TL_Gain''),else, web([''jar:file:///'',matlabroot,''/help/toolbox/simulink/help.jar!/slref/' lower(get_param(gcbh,'Blocktype')) '.html''], ''-helpbrowser''),end'])
      mask Display: plot([0, .9, 0],[.05, .5, .95])
  Gain1 : Gain  RequirementInfo={} %GIDa_aeb3c446_d0b6_483a_af00_9b33d2f615c7  OutDataTypeStr=int32  mask(TL_Gain){data={'output',{'type','Int32'},'date',735951.66839809029}}
      settings: CopyFcn=if exist('tl_reset_reviewflag','file')==2,tl_reset_reviewflag(gcbh);end  DeleteFcn=if exist('delete_tlblock','file')==2,delete_tlblock(gcbh);end  NameChangeFcn=if exist('rename_tlblock','file')==2,rename_tlblock(gcbh);end  OpenFcn=if exist('tl_open_blockdlg','file')==2,tl_open_blockdlg(gcbh);else,open_system(gcbh,'parameter');end
      mask Help: eval(['if exist(''tl_online_help'',''file'') == 2, tl_online_help(''Topic'',''TL_Gain''),else, web([''jar:file:///'',matlabroot,''/help/toolbox/simulink/help.jar!/slref/' lower(get_param(gcbh,'Blocktype')) '.html''], ''-helpbrowser''),end'])
      mask Display: plot([0, .9, 0],[.05, .5, .95])
  If : If  RequirementInfo={} %GIDa_7f209655_7e19_44a9_aa13_f300246fca54  IfExpression=u1
  Logical Operator : Logic  RequirementInfo={} %GIDa_929e8ded_97ba_4dd9_af32_0236d5c2f995  Operator=NOT  Inputs=1  AllPortsSameDT=off  OutDataTypeStr=boolean  mask(TL_LogicalOperator){data={'date',735951.66839760414}}
      settings: DeleteFcn=if exist('delete_tlblock','file')==2,delete_tlblock(gcbh);end  NameChangeFcn=if exist('rename_tlblock','file')==2,rename_tlblock(gcbh);end  OpenFcn=if exist('tl_open_blockdlg','file')==2,tl_open_blockdlg(gcbh);else,open_system(gcbh,'parameter');end
      mask Help: eval(['if exist(''tl_online_help'',''file'') == 2, tl_online_help(''Topic'',''TL_LogicalOperator''),else, web([''jar:file:///'',matlabroot,''/help/toolbox/simulink/help.jar!/slref/' lower(get_param(gcbh,'Blocktype')) '.html''], ''-helpbrowser''),end'])
      mask Display: plot([-0.05, 1.05, NaN, -0.05, 1.05],[.01, .01, NaN, .99, .99])
  Logical Operator1 : Logic  RequirementInfo={} %GIDa_9913b8d9_e522_4a40_85e7_0a54b56de6e2  Operator=NOT  Inputs=1  AllPortsSameDT=off  OutDataTypeStr=boolean  mask(TL_LogicalOperator){data={'date',735951.66839734954}}
      settings: DeleteFcn=if exist('delete_tlblock','file')==2,delete_tlblock(gcbh);end  NameChangeFcn=if exist('rename_tlblock','file')==2,rename_tlblock(gcbh);end  OpenFcn=if exist('tl_open_blockdlg','file')==2,tl_open_blockdlg(gcbh);else,open_system(gcbh,'parameter');end
      mask Help: eval(['if exist(''tl_online_help'',''file'') == 2, tl_online_help(''Topic'',''TL_LogicalOperator''),else, web([''jar:file:///'',matlabroot,''/help/toolbox/simulink/help.jar!/slref/' lower(get_param(gcbh,'Blocktype')) '.html''], ''-helpbrowser''),end'])
      mask Display: plot([-0.05, 1.05, NaN, -0.05, 1.05],[.01, .01, NaN, .99, .99])
  Logical Operator2 : Logic  RequirementInfo={} %GIDa_24d52867_87f8_4dc4_8c8c_37d868352cf5  AllPortsSameDT=off  OutDataTypeStr=boolean  mask(TL_LogicalOperator){data={'date',735951.66839709494}}
      settings: DeleteFcn=if exist('delete_tlblock','file')==2,delete_tlblock(gcbh);end  NameChangeFcn=if exist('rename_tlblock','file')==2,rename_tlblock(gcbh);end  OpenFcn=if exist('tl_open_blockdlg','file')==2,tl_open_blockdlg(gcbh);else,open_system(gcbh,'parameter');end
      mask Help: eval(['if exist(''tl_online_help'',''file'') == 2, tl_online_help(''Topic'',''TL_LogicalOperator''),else, web([''jar:file:///'',matlabroot,''/help/toolbox/simulink/help.jar!/slref/' lower(get_param(gcbh,'Blocktype')) '.html''], ''-helpbrowser''),end'])
      mask Display: plot([-0.05, 1.05, NaN, -0.05, 1.05],[.01, .01, NaN, .99, .99])
  Merge : Merge  RequirementInfo={} %GIDa_9a536079_948b_4fea_b746_469d2b14d2cb  InitialOutput=0  mask(TL_Merge){data={'output',{'inheritscaling',0},'date',735951.6683968287}}
      settings: CopyFcn=if exist('tl_reset_reviewflag','file')==2,tl_reset_reviewflag(gcbh);end  DeleteFcn=if exist('delete_tlblock','file')==2,delete_tlblock(gcbh);end  NameChangeFcn=if exist('rename_tlblock','file')==2,rename_tlblock(gcbh);end  OpenFcn=if exist('tl_open_blockdlg','file')==2,tl_open_blockdlg(gcbh);else,open_system(gcbh,'parameter');end
      mask Help: eval(['if exist(''tl_online_help'',''file'') == 2, tl_online_help(''Topic'',''TL_Merge''),else, web([''jar:file:///'',matlabroot,''/help/toolbox/simulink/help.jar!/slref/' lower(get_param(gcbh,'Blocktype')) '.html''], ''-helpbrowser''),end'])
      mask Display: plot([-0.05, 1.05, NaN, -0.05, 1.05],[.01, .01, NaN, .99, .99])
  Merge1 : Merge  RequirementInfo={} %GIDa_6a221547_98d7_4f84_8de9_428e28441ee4  InitialOutput=0  mask(TL_Merge){data={'output',{'type','Int32','inheritscaling',0},'date',735951.66839645838}}
      settings: CopyFcn=if exist('tl_reset_reviewflag','file')==2,tl_reset_reviewflag(gcbh);end  DeleteFcn=if exist('delete_tlblock','file')==2,delete_tlblock(gcbh);end  NameChangeFcn=if exist('rename_tlblock','file')==2,rename_tlblock(gcbh);end  OpenFcn=if exist('tl_open_blockdlg','file')==2,tl_open_blockdlg(gcbh);else,open_system(gcbh,'parameter');end
      mask Help: eval(['if exist(''tl_online_help'',''file'') == 2, tl_online_help(''Topic'',''TL_Merge''),else, web([''jar:file:///'',matlabroot,''/help/toolbox/simulink/help.jar!/slref/' lower(get_param(gcbh,'Blocktype')) '.html''], ''-helpbrowser''),end'])
      mask Display: plot([-0.05, 1.05, NaN, -0.05, 1.05],[.01, .01, NaN, .99, .99])
  PID Regulation : Subsystem  RequirementInfo={} %GIDa_b2c2dc06_4b83_4e6b_82c9_df95dc5bf194  TreatAsAtomicUnit=on
  Standard Regulation : Subsystem  RequirementInfo={} %GIDa_4e9f5b64_2272_48f9_b7aa_b4c7cd676117  TreatAsAtomicUnit=on
  s16UnsaturatedMoterPowerOrder : Outport  RequirementInfo={} %GIDa_52833ac1_593d_4975_83bc_81047b817c76  InitialOutput=0
  s32IntegerError : Outport  RequirementInfo={} %GIDa_33a2a037_9ada_46ce_b46f_1b94ba6dedbf  Port=2  InitialOutput=0
  wires:
  Logical Operator/1 -> Logical Operator2/1
  Logical Operator1/1 -> Logical Operator2/2
  bIsPIDMotor/1 -> Logical Operator/1, PID Regulation/1(bIsPIDMotor)
  bIsPIDSupply/1 -> Logical Operator1/1, PID Regulation/2(bIsPIDSupply)
  If/1 -> Standard Regulation/Action
  Logical Operator2/1 -> If/1
  Standard Regulation/1(sUnsaturatedMotorPowerOrder) -> Merge/1
  Merge/1 -> Gain/1
  s32OrderToApply/1 -> PID Regulation/3(s32OrderToApply), Standard Regulation/1(s32MilliOrderToApply)
  bIsNewCycle/1 -> Standard Regulation/2(bIsNewProfile)
  If/2 -> PID Regulation/Action
  PID Regulation/1(s16UnsaturatedMotorPowerOrder) -> Merge/2
  u32MeasuredCurrent/1 -> PID Regulation/4(u32MeasuredCurrent), Standard Regulation/3(u32MeasuredCurrentIn_mA)
  s16OldPWM/1 -> PID Regulation/5(s16OldPWM), Standard Regulation/5(s16OldPWM)
  u16BatteryVoltage/1 -> PID Regulation/6(u16BatteryVoltage), Standard Regulation/7(u16BatteryVoltage)
  Gain/1 -> s16UnsaturatedMoterPowerOrder/1
  s32OldErrorInteger/1 -> PID Regulation/7(s32OldErrorInteger), Standard Regulation/6(s32OldErrorInteger)
  Merge1/1 -> Gain1/1
  Gain1/1 -> s32IntegerError/1
  PID Regulation/2(s32IntegerError) -> Merge1/2
  Standard Regulation/2(s32IntegerError) -> Merge1/1
  bIsNewStepBegin/1 -> Standard Regulation/4(bIsNewStepBegin)
